simulink model "BrushlessDCMotor"  (R2023b)
settings: Solver=VariableStepAuto  StartTime=0.0  StopTime=10.0  RelTol=1e-3
libraries: autolibbldc x1, eeBldcCommutationLogic x1
settings Model: Creator=jwilson  LastModifiedBy=jwilson

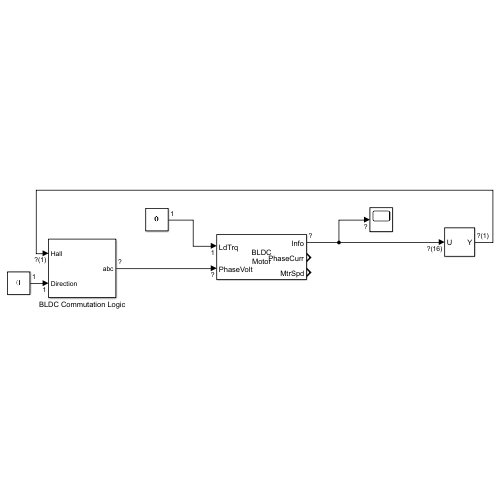
[thumbnail: Simulink's stored preview of the top-level diagram]
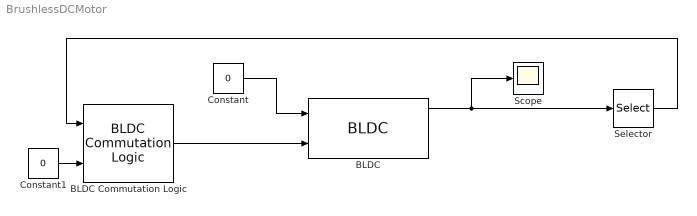
== system BrushlessDCMotor ==
  BLDC : autolibbldc/BLDC  VariantControl=pmsmVariant==pmsmEnum.TorqueInput  MechInput=Torque  SimType=Continuous  BlockSampleTime=25e-6  p=4  Rs=0.36  Ld=2e-4  Lq=2e-4  Lambda=0.0064  J=7.0616e-06  B=2.6369e-06  F=0  Id_init=0  Iq_init=0  Th_init=0  Omega_init=0  RefBlkName='autolibbldc/BLDC'  aMode=5
      settings: LibrarySourceBlock=mcblib/Electrical Systems/Motors/BLDC
  BLDC Commutation Logic : eeBldcCommutationLogic/BLDC Commutation Logic  Ts=-1
      settings: LibrarySourceBlock=ee_sl_lib/BLDC Control/BLDC Commutation Logic
  Constant : Constant  Value=0
  Constant1 : Constant  Value=0
  Scope : Scope
  Selector : Selector  InputPortWidth=16  IndexOptions=Index vector (dialog)  Indices=[16]  OutputSizes=1
  wires:
  BLDC Commutation Logic/1 -> BLDC/2
  BLDC/1 -> Selector/1, Scope/1
  Constant/1 -> BLDC/1
  Constant1/1 -> BLDC Commutation Logic/2
  Selector/1 -> BLDC Commutation Logic/1
